simulink model "bit32alu"  (R2020a)
settings: Solver=VariableStepAuto  StartTime=0.0  StopTime=10.0  RelTol=1e-3
(part 1 of 62)
settings Model: Creator=kishan  LastModifiedBy=kishan

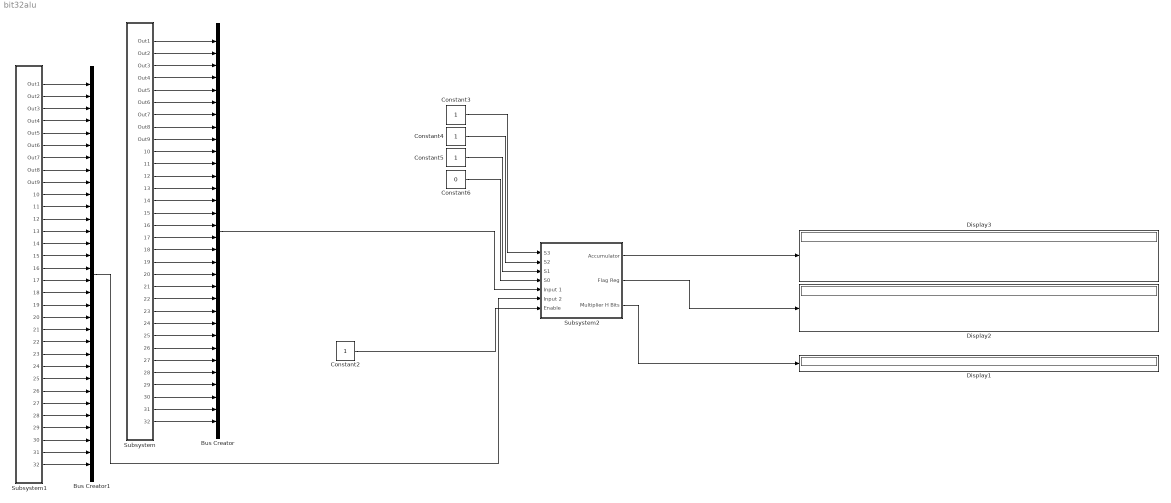
== system bit32alu ==
  Bus Creator : BusCreator  Inputs=32
  Bus Creator1 : BusCreator  Inputs=32
  Constant{2..5} (4 alike) : Constant  OutDataTypeStr=boolean
  Constant6 : Constant  Value=0  OutDataTypeStr=boolean
  Display1 : Display
  Display2 : Display
  Display3 : Display
  Subsystem : Subsystem
  Subsystem1 : Subsystem
  Subsystem2 : Subsystem
  wires:
  Subsystem/2(Out2) -> Bus Creator/2
  Subsystem/30(Out30) -> Bus Creator/30
  Subsystem/31(Out31) -> Bus Creator/31
  Subsystem/11(Out11) -> Bus Creator/11
  Subsystem/26(Out26) -> Bus Creator/26
  Subsystem/9(Out9) -> Bus Creator/9
  Subsystem/17(Out17) -> Bus Creator/17
  Subsystem/27(Out27) -> Bus Creator/27
  Subsystem/32(Out32) -> Bus Creator/32
  Subsystem/7(Out7) -> Bus Creator/7
  Subsystem/16(Out16) -> Bus Creator/16
  Subsystem/25(Out25) -> Bus Creator/25
  Subsystem/15(Out15) -> Bus Creator/15
  Subsystem/22(Out22) -> Bus Creator/22
  Subsystem/23(Out23) -> Bus Creator/23
  Subsystem/10(Out10) -> Bus Creator/10
  Subsystem/12(Out12) -> Bus Creator/12
  Subsystem/13(Out13) -> Bus Creator/13
  Subsystem/20(Out20) -> Bus Creator/20
  Subsystem/29(Out29) -> Bus Creator/29
  Subsystem/3(Out3) -> Bus Creator/3
  Subsystem/4(Out4) -> Bus Creator/4
  Subsystem/6(Out6) -> Bus Creator/6
  Subsystem/24(Out24) -> Bus Creator/24
  Subsystem/18(Out18) -> Bus Creator/18
  Subsystem/1(Out1) -> Bus Creator/1
  Subsystem/28(Out28) -> Bus Creator/28
  Subsystem/14(Out14) -> Bus Creator/14
  Subsystem/8(Out8) -> Bus Creator/8
  Subsystem/5(Out5) -> Bus Creator/5
  Subsystem/21(Out21) -> Bus Creator/21
  Subsystem/19(Out19) -> Bus Creator/19
  Subsystem1/2(Out2) -> Bus Creator1/2
  Subsystem1/30(Out30) -> Bus Creator1/30
  Subsystem1/31(Out31) -> Bus Creator1/31
  Subsystem1/11(Out11) -> Bus Creator1/11
  Subsystem1/26(Out26) -> Bus Creator1/26
  Subsystem1/9(Out9) -> Bus Creator1/9
  Subsystem1/17(Out17) -> Bus Creator1/17
  Subsystem1/27(Out27) -> Bus Creator1/27
  Subsystem1/32(Out32) -> Bus Creator1/32
  Subsystem1/7(Out7) -> Bus Creator1/7
  Subsystem1/16(Out16) -> Bus Creator1/16
  Subsystem1/25(Out25) -> Bus Creator1/25
  Subsystem1/15(Out15) -> Bus Creator1/15
  Subsystem1/22(Out22) -> Bus Creator1/22
  Subsystem1/23(Out23) -> Bus Creator1/23
  Subsystem1/10(Out10) -> Bus Creator1/10
  Subsystem1/12(Out12) -> Bus Creator1/12
  Subsystem1/13(Out13) -> Bus Creator1/13
  Subsystem1/20(Out20) -> Bus Creator1/20
  Subsystem1/29(Out29) -> Bus Creator1/29
  Subsystem1/3(Out3) -> Bus Creator1/3
  Subsystem1/4(Out4) -> Bus Creator1/4
  Subsystem1/6(Out6) -> Bus Creator1/6
  Subsystem1/24(Out24) -> Bus Creator1/24
  Subsystem1/18(Out18) -> Bus Creator1/18
  Subsystem1/1(Out1) -> Bus Creator1/1
  Subsystem1/28(Out28) -> Bus Creator1/28
  Subsystem1/14(Out14) -> Bus Creator1/14
  Subsystem1/8(Out8) -> Bus Creator1/8
  Subsystem1/5(Out5) -> Bus Creator1/5
  Subsystem1/21(Out21) -> Bus Creator1/21
  Subsystem1/19(Out19) -> Bus Creator1/19
  Constant3/1 -> Subsystem2/1(S3)
  Constant4/1 -> Subsystem2/2(S2)
  Constant5/1 -> Subsystem2/3(S1)
  Constant6/1 -> Subsystem2/4(S0)
  Bus Creator/1 -> Subsystem2/5(Input 1)
  Bus Creator1/1 -> Subsystem2/6(Input 2)
  Constant2/1 -> Subsystem2/7(Enable)
  Subsystem2/1(Accumulator) -> Display3/1
  Subsystem2/2(Flag Reg) -> Display2/1
  Subsystem2/3(Multiplier H Bits) -> Display1/1

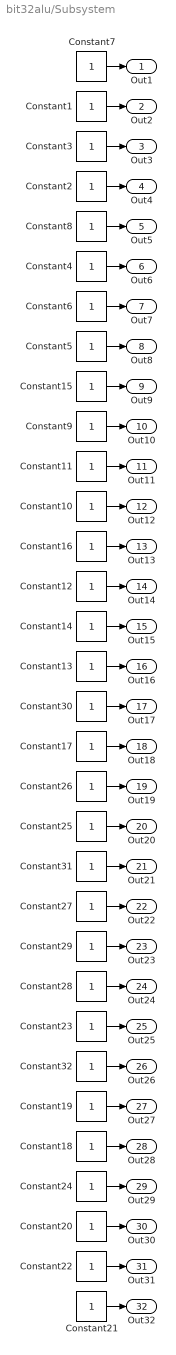
== system bit32alu/Subsystem ==
  Constant{1..32} (32 alike) : Constant  OutDataTypeStr=boolean
  Out1 : Outport
  Out2 : Outport  Port=2
  Out3 : Outport  Port=3
  Out4 : Outport  Port=4
  Out5 : Outport  Port=5
  Out6 : Outport  Port=6
  Out7 : Outport  Port=7
  Out8 : Outport  Port=8
  Out9 : Outport  Port=9
  Out10 : Outport  Port=10
  Out11 : Outport  Port=11
  Out12 : Outport  Port=12
  Out13 : Outport  Port=13
  Out14 : Outport  Port=14
  Out15 : Outport  Port=15
  Out16 : Outport  Port=16
  Out17 : Outport  Port=17
  Out18 : Outport  Port=18
  Out19 : Outport  Port=19
  Out20 : Outport  Port=20
  Out21 : Outport  Port=21
  Out22 : Outport  Port=22
  Out23 : Outport  Port=23
  Out24 : Outport  Port=24
  Out25 : Outport  Port=25
  Out26 : Outport  Port=26
  Out27 : Outport  Port=27
  Out28 : Outport  Port=28
  Out29 : Outport  Port=29
  Out30 : Outport  Port=30
  Out31 : Outport  Port=31
  Out32 : Outport  Port=32
  wires:
  Constant7/1 -> Out1/1
  Constant1/1 -> Out2/1
  Constant3/1 -> Out3/1
  Constant2/1 -> Out4/1
  Constant8/1 -> Out5/1
  Constant5/1 -> Out8/1
  Constant4/1 -> Out6/1
  Constant6/1 -> Out7/1
  Constant15/1 -> Out9/1
  Constant13/1 -> Out16/1
  Constant12/1 -> Out14/1
  Constant16/1 -> Out13/1
  Constant10/1 -> Out12/1
  Constant9/1 -> Out10/1
  Constant14/1 -> Out15/1
  Constant11/1 -> Out11/1
  Constant24/1 -> Out29/1
  Constant23/1 -> Out25/1
  Constant19/1 -> Out27/1
  Constant25/1 -> Out20/1
  Constant31/1 -> Out21/1
  Constant30/1 -> Out17/1
  Constant22/1 -> Out31/1
  Constant28/1 -> Out24/1
  Constant29/1 -> Out23/1
  Constant27/1 -> Out22/1
  Constant21/1 -> Out32/1
  Constant26/1 -> Out19/1
  Constant18/1 -> Out28/1
  Constant17/1 -> Out18/1
  Constant20/1 -> Out30/1
  Constant32/1 -> Out26/1

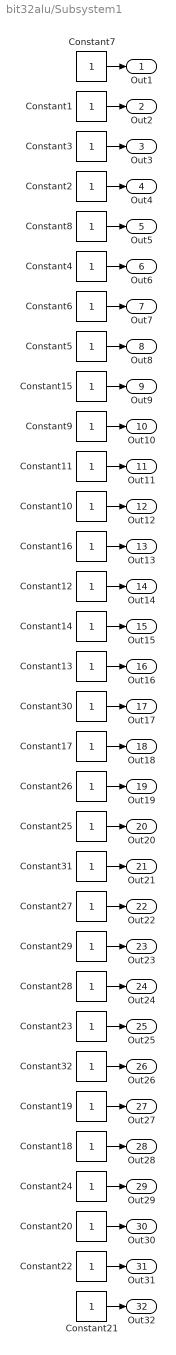
== system bit32alu/Subsystem1 ==
  Constant{1..32} (32 alike) : Constant  OutDataTypeStr=boolean
  Out1 : Outport
  Out2 : Outport  Port=2
  Out3 : Outport  Port=3
  Out4 : Outport  Port=4
  Out5 : Outport  Port=5
  Out6 : Outport  Port=6
  Out7 : Outport  Port=7
  Out8 : Outport  Port=8
  Out9 : Outport  Port=9
  Out10 : Outport  Port=10
  Out11 : Outport  Port=11
  Out12 : Outport  Port=12
  Out13 : Outport  Port=13
  Out14 : Outport  Port=14
  Out15 : Outport  Port=15
  Out16 : Outport  Port=16
  Out17 : Outport  Port=17
  Out18 : Outport  Port=18
  Out19 : Outport  Port=19
  Out20 : Outport  Port=20
  Out21 : Outport  Port=21
  Out22 : Outport  Port=22
  Out23 : Outport  Port=23
  Out24 : Outport  Port=24
  Out25 : Outport  Port=25
  Out26 : Outport  Port=26
  Out27 : Outport  Port=27
  Out28 : Outport  Port=28
  Out29 : Outport  Port=29
  Out30 : Outport  Port=30
  Out31 : Outport  Port=31
  Out32 : Outport  Port=32
  wires:
  Constant7/1 -> Out1/1
  Constant1/1 -> Out2/1
  Constant3/1 -> Out3/1
  Constant2/1 -> Out4/1
  Constant8/1 -> Out5/1
  Constant5/1 -> Out8/1
  Constant4/1 -> Out6/1
  Constant6/1 -> Out7/1
  Constant15/1 -> Out9/1
  Constant13/1 -> Out16/1
  Constant12/1 -> Out14/1
  Constant16/1 -> Out13/1
  Constant10/1 -> Out12/1
  Constant9/1 -> Out10/1
  Constant14/1 -> Out15/1
  Constant11/1 -> Out11/1
  Constant24/1 -> Out29/1
  Constant23/1 -> Out25/1
  Constant19/1 -> Out27/1
  Constant25/1 -> Out20/1
  Constant31/1 -> Out21/1
  Constant30/1 -> Out17/1
  Constant22/1 -> Out31/1
  Constant28/1 -> Out24/1
  Constant29/1 -> Out23/1
  Constant27/1 -> Out22/1
  Constant21/1 -> Out32/1
  Constant26/1 -> Out19/1
  Constant18/1 -> Out28/1
  Constant17/1 -> Out18/1
  Constant20/1 -> Out30/1
  Constant32/1 -> Out26/1

== system bit32alu/Subsystem2 ==
  S3 : Inport
  S2 : Inport  Port=2
  S1 : Inport  Port=3
  S0 : Inport  Port=4
  Input 1 : Inport  Port=5
  Input 2 : Inport  Port=6
  Enable : Inport  Port=7
  Adder : Subsystem
  Comparartor : Subsystem
  Decrementer : Subsystem
  Demux : Demux  Outputs=32
  Demux1 : Demux  Outputs=32
  Incrementer : Subsystem
  Left Rotator : Subsystem
  Left shifter : Subsystem
  Logical Operator : Logic  AllPortsSameDT=off  OutDataTypeStr=boolean
  Logical Operator1 : Logic  Operator=OR  AllPortsSameDT=off  OutDataTypeStr=boolean
  Logical Operator2 : Logic  Operator=NOT  AllPortsSameDT=off  OutDataTypeStr=boolean
  Logical Operator4 : Logic  Operator=NOR  Inputs=32  AllPortsSameDT=off  OutDataTypeStr=boolean
  Logical Operator5 : Logic  Operator=NXOR  Inputs=32  AllPortsSameDT=off  OutDataTypeStr=boolean
  Multiplier : Subsystem
  Mux : Mux  Inputs=8
  Ones : Constant  Value=[1 1 1 1 1 1 1 1 1 1 1 1 1 1 1 1 1 1 1 1 1 1 1 1 1 1 1 1 1 1 1 1]  OutDataTypeStr=boolean
  Right Shifter : Subsystem
  Right rotator : Subsystem
  Subsystem7 : Subsystem
  Subtractor : Subsystem
  Zeros : Constant  Value=[0 0 0 0 0 0 0 0 0 0 0 0 0 0 0 0 0 0 0 0 0 0 0 0 0 0 0 0 0 0 0 0]  OutDataTypeStr=boolean
  Accumulator : Outport
  Flag Reg : Outport  Port=2
  Multiplier H Bits : Outport  Port=3
  wires:
  Demux1/11 -> Logical Operator5/11
  Demux/9 -> Logical Operator4/9
  Demux/26 -> Logical Operator4/26
  Demux1/3 -> Logical Operator5/3
  Demux/12 -> Logical Operator4/12
  Demux1/16 -> Logical Operator5/16
  Demux/32 -> Logical Operator4/32
  Demux/14 -> Logical Operator4/14
  Demux/28 -> Logical Operator4/28
  Demux1/14 -> Logical Operator5/14
  Left Rotator/1(Out4) -> Subsystem7/17(In17)
  Demux1/13 -> Logical Operator5/13
  Demux/2 -> Logical Operator4/2
  S2/1 -> Subsystem7/2(In3)
  Right Shifter/2(Out4) -> Subsystem7/13(In13)
  Enable/1 -> Subsystem7/21(In21)
  Demux1/22 -> Logical Operator5/22
  Demux1/32 -> Logical Operator5/32
  Demux1/6 -> Logical Operator5/6
  Comparartor/1(Out1) -> Subsystem7/20(In20)
  Demux1/18 -> Logical Operator5/18
  Subsystem7/1(Out1) -> Accumulator/1, Demux1/1, Demux/1
  Demux/5 -> Logical Operator4/5
  Logical Operator1/1 -> Subsystem7/8(In6)
  Demux/11 -> Logical Operator4/11
  S3/1 -> Subsystem7/1(In1)
  Mux/1 -> Flag Reg/1
  Adder/1(Out1) -> Mux/5
  Logical Operator/1 -> Subsystem7/7(In4)
  Demux/31 -> Logical Operator4/31
  Logical Operator4/1 -> Mux/7
  Demux1/30 -> Logical Operator5/30
  Subtractor/1(Out1) -> Mux/6
  Demux/23 -> Logical Operator4/23
  Ones/1 -> Subsystem7/6(In2)
  Logical Operator5/1 -> Mux/8
  Demux/22 -> Logical Operator4/22
  Adder/2(Out2) -> Subsystem7/14(In14)
  Subtractor/2(Out2) -> Subsystem7/15(In15)
  Decrementer/2(Out2) -> Subsystem7/12(In12)
  Demux1/17 -> Logical Operator5/17
  Demux/6 -> Logical Operator4/6
  Demux/4 -> Logical Operator4/4
  Right rotator/1(Out2) -> Subsystem7/18(In18)
  Demux1/9 -> Logical Operator5/9
  Right Shifter/1(Out3) -> Mux/4
  Demux/17 -> Logical Operator4/17
  Demux/15 -> Logical Operator4/15
  Demux/7 -> Logical Operator4/7
  Demux1/2 -> Logical Operator5/2
  Demux1/5 -> Logical Operator5/5
  Demux1/31 -> Logical Operator5/31
  Zeros/1 -> Subsystem7/5(In9)
  Input 1/1 -> Left Rotator/1(Input 1), Right rotator/1(Input 1), Comparartor/1(In1), Adder/1(In1), Subsystem7/16(Input 1), Left shifter/1(Input 1), Right Shifter/1(Input 1), Decrementer/1(In1), Incrementer/1(In1), Logical Operator2/1, Logical Operator/1, Logical Operator1/1, Subtractor/1(In1), Multiplier/1(In1)
  Multiplier/2(Out2) -> Subsystem7/19(In19)
  Left shifter/1(Out1) -> Mux/2
  Demux1/27 -> Logical Operator5/27
  Demux/30 -> Logical Operator4/30
  Demux1/21 -> Logical Operator5/21
  Demux/18 -> Logical Operator4/18
  Demux/21 -> Logical Operator4/21
  Demux1/20 -> Logical Operator5/20
  Demux1/28 -> Logical Operator5/28
  Demux1/10 -> Logical Operator5/10
  Demux1/25 -> Logical Operator5/25
  Demux/29 -> Logical Operator4/29
  Incrementer/2(Out2) -> Subsystem7/10(In10)
  Left shifter/2(Out2) -> Subsystem7/11(In11)
  Demux/20 -> Logical Operator4/20
  Demux1/19 -> Logical Operator5/19
  Demux1/8 -> Logical Operator5/8
  Demux/25 -> Logical Operator4/25
  Demux1/1 -> Logical Operator5/1
  Demux1/15 -> Logical Operator5/15
  Demux1/23 -> Logical Operator5/23
  Multiplier/1(Out1) -> Multiplier H Bits/1
  Demux/8 -> Logical Operator4/8
  Demux/1 -> Logical Operator4/1
  Demux1/26 -> Logical Operator5/26
  Demux1/24 -> Logical Operator5/24
  S0/1 -> Subsystem7/4(In7)
  Logical Operator2/1 -> Subsystem7/9(In8)
  Demux/10 -> Logical Operator4/10
  Demux/24 -> Logical Operator4/24
  Decrementer/1(Out1) -> Mux/3
  Demux1/4 -> Logical Operator5/4
  Demux/16 -> Logical Operator4/16
  Demux1/12 -> Logical Operator5/12
  Demux/3 -> Logical Operator4/3
  Incrementer/1(Out1) -> Mux/1
  Demux1/7 -> Logical Operator5/7
  Demux/13 -> Logical Operator4/13
  Input 2/1 -> Comparartor/2(In2), Logical Operator1/2, Logical Operator/2, Subtractor/2(In2), Adder/2(In2), Multiplier/2(In2)
  Demux/19 -> Logical Operator4/19
  Demux/27 -> Logical Operator4/27
  S1/1 -> Subsystem7/3(In5)
  Demux1/29 -> Logical Operator5/29

== system bit32alu/Subsystem2/Adder ==
  In1 : Inport
  In2 : Inport  Port=2
  Subsystem : Subsystem
  Zeros1 : Constant  Value=0  OutDataTypeStr=boolean
  Out1 : Outport
  Out2 : Outport  Port=2
  wires:
  Subsystem/2(Out2) -> Out2/1
  In2/1 -> Subsystem/3(In3)
  Zeros1/1 -> Subsystem/2(In2)
  In1/1 -> Subsystem/1(In1)
  Subsystem/1(Out1) -> Out1/1

== system bit32alu/Subsystem2/Comparartor ==
  In1 : Inport
  In2 : Inport  Port=2
  Comparator : Subsystem
  Comparator1 : Subsystem
  Comparator2 : Subsystem
  Comparator3 : Subsystem
  Demux : Demux
  Demux1 : Demux
  Display : Display
  Logical Operator : Logic  Operator=OR  Inputs=4  AllPortsSameDT=off  OutDataTypeStr=boolean
  Logical Operator1 : Logic  Inputs=4  AllPortsSameDT=off  OutDataTypeStr=boolean
  Logical Operator2 : Logic  AllPortsSameDT=off  OutDataTypeStr=boolean
  Logical Operator3 : Logic  Inputs=3  AllPortsSameDT=off  OutDataTypeStr=boolean
  Logical Operator4 : Logic  Inputs=4  AllPortsSameDT=off  OutDataTypeStr=boolean
  Logical Operator5 : Logic  Operator=NOR  AllPortsSameDT=off  OutDataTypeStr=boolean
  Mux : Mux
  Mux1 : Mux
  Zeros1 : Constant  Value=[0 0 0 0 0 0 0 0 0 0 0 0 0 0 0 0 0 0 0 0 0 0 0 0 0 0 0 0 0]  OutDataTypeStr=boolean
  Out1 : Outport
  wires:
  Zeros1/1 -> Mux/4
  Mux/1 -> Out1/1
  In1/1 -> Demux/1
  In2/1 -> Demux1/1
  Demux/1 -> Comparator/1(In1)
  Demux/2 -> Comparator1/1(In1)
  Demux/3 -> Comparator2/1(In1)
  Demux/4 -> Comparator3/1(In1)
  Demux1/1 -> Comparator/2(In2)
  Demux1/2 -> Comparator1/2(In2)
  Demux1/3 -> Comparator2/2(In2)
  Demux1/4 -> Comparator3/2(In2)
  Comparator/2(Out2) -> Logical Operator1/1, Logical Operator4/1, Logical Operator3/1, Logical Operator2/1
  Comparator1/2(Out2) -> Logical Operator4/2, Logical Operator3/2, Logical Operator1/2
  Comparator2/2(Out2) -> Logical Operator4/3, Logical Operator1/3
  Comparator3/2(Out2) -> Logical Operator1/4
  Logical Operator1/1 -> Logical Operator5/2, Mux/2
  Mux1/1 -> Display/1
  Comparator/1(Out1) -> Logical Operator/1
  Comparator1/1(Out1) -> Logical Operator2/2
  Logical Operator2/1 -> Logical Operator/2
  Comparator2/1(Out1) -> Logical Operator3/3
  Logical Operator3/1 -> Logical Operator/3
  Comparator3/1(Out1) -> Logical Operator4/4
  Logical Operator4/1 -> Logical Operator/4
  Logical Operator/1 -> Logical Operator5/1, Mux/1
  Comparator/3(Out3) -> Mux1/1
  Comparator1/3(Out3) -> Mux1/2
  Comparator2/3(Out3) -> Mux1/3
  Comparator3/3(Out3) -> Mux1/4
  Logical Operator5/1 -> Mux/3

== system bit32alu/Subsystem2/Decrementer ==
  In1 : Inport
  Subtractor1 : Subsystem
  Zeros1 : Constant  Value=[0 0 0 0 0 0 0 0 0 0 0 0 0 0 0 0 0 0 0 0 0 0 0 0 0 0 0 0 0 0 0 1]
  Out1 : Outport
  Out2 : Outport  Port=2
  wires:
  Zeros1/1 -> Subtractor1/2(In2)
  In1/1 -> Subtractor1/1(In1)
  Subtractor1/1(Out1) -> Out1/1
  Subtractor1/2(Out2) -> Out2/1

== system bit32alu/Subsystem2/Incrementer ==
  In1 : Inport
  Incrementer : Subsystem
  Zeros1 : Constant  Value=[0 0 0 0 0 0 0 0 0 0 0 0 0 0 0 0 0 0 0 0 0 0 0 0 0 0 0 0 0 0 0 1]  OutDataTypeStr=boolean
  Out1 : Outport
  Out2 : Outport  Port=2
  wires:
  Zeros1/1 -> Incrementer/2(In2)
  In1/1 -> Incrementer/1(In1)
  Incrementer/2(Out2) -> Out2/1
  Incrementer/1(Out1) -> Out1/1

== system bit32alu/Subsystem2/Left Rotator ==
  Input 1 : Inport
  Demux : Demux  Outputs=32
  Mux : Mux  Inputs=32
  Out4 : Outport
  wires:
  Input 1/1 -> Demux/1
  Mux/1 -> Out4/1
  Demux/1 -> Mux/2
  Demux/2 -> Mux/3
  Demux/3 -> Mux/4
  Demux/4 -> Mux/5
  Demux/5 -> Mux/6
  Demux/6 -> Mux/7
  Demux/7 -> Mux/8
  Demux/8 -> Mux/9
  Demux/9 -> Mux/10
  Demux/10 -> Mux/11
  Demux/11 -> Mux/12
  Demux/12 -> Mux/13
  Demux/13 -> Mux/14
  Demux/14 -> Mux/15
  Demux/15 -> Mux/16
  Demux/16 -> Mux/17
  Demux/17 -> Mux/18
  Demux/18 -> Mux/19
  Demux/19 -> Mux/20
  Demux/20 -> Mux/21
  Demux/21 -> Mux/22
  Demux/22 -> Mux/23
  Demux/23 -> Mux/24
  Demux/24 -> Mux/25
  Demux/25 -> Mux/26
  Demux/26 -> Mux/27
  Demux/27 -> Mux/28
  Demux/28 -> Mux/29
  Demux/29 -> Mux/30
  Demux/30 -> Mux/31
  Demux/31 -> Mux/32
  Demux/32 -> Mux/1

== system bit32alu/Subsystem2/Left shifter ==
  Input 1 : Inport
  Demux : Demux  Outputs=32
  Mux : Mux  Inputs=32
  Zeros1 : Constant  Value=0  OutDataTypeStr=boolean
  Out1 : Outport
  Out2 : Outport  Port=2
  wires:
  Zeros1/1 -> Mux/32
  Input 1/1 -> Demux/1
  Mux/1 -> Out2/1
  Demux/1 -> Out1/1
  Demux/2 -> Mux/1
  Demux/3 -> Mux/2
  Demux/4 -> Mux/3
  Demux/5 -> Mux/4
  Demux/6 -> Mux/5
  Demux/7 -> Mux/6
  Demux/8 -> Mux/7
  Demux/9 -> Mux/8
  Demux/10 -> Mux/9
  Demux/11 -> Mux/10
  Demux/12 -> Mux/11
  Demux/13 -> Mux/12
  Demux/14 -> Mux/13
  Demux/15 -> Mux/14
  Demux/16 -> Mux/15
  Demux/17 -> Mux/16
  Demux/18 -> Mux/17
  Demux/19 -> Mux/18
  Demux/20 -> Mux/19
  Demux/21 -> Mux/20
  Demux/22 -> Mux/21
  Demux/23 -> Mux/22
  Demux/24 -> Mux/23
  Demux/25 -> Mux/24
  Demux/26 -> Mux/25
  Demux/27 -> Mux/26
  Demux/28 -> Mux/27
  Demux/29 -> Mux/28
  Demux/30 -> Mux/29
  Demux/31 -> Mux/30
  Demux/32 -> Mux/31

== system bit32alu/Subsystem2/Multiplier ==
  In1 : Inport
  In2 : Inport  Port=2
  Constant : Constant  Value=0  OutDataTypeStr=boolean
  Constant1 : Constant  Value=0  OutDataTypeStr=boolean
  Constant2 : Constant  Value=[0 0 0 0 0 0 0 0 0 0 0 0 0 0 0]  OutDataTypeStr=boolean
  Demux : Demux  Outputs=2
  Demux1 : Demux  Outputs=2
  Demux2 : Demux  Outputs=2
  Display : Display
  Logical Operator : Logic  AllPortsSameDT=off  OutDataTypeStr=boolean
  Logical Operator1 : Logic  Operator=XOR  AllPortsSameDT=off  OutDataTypeStr=boolean
  Mux{,1..3} (4 alike) : Mux  Inputs=2
  Mux4 : Mux  Inputs=3
  Subsystem : Subsystem
  Subsystem1 : Subsystem
  Subsystem2 : Subsystem
  Subsystem3 : Subsystem
  Subsystem4 : Subsystem
  Subsystem5 : Subsystem
  Subsystem7 : Subsystem
  Out1 : Outport
  Out2 : Outport  Port=2
  wires:
  Constant1/1 -> Subsystem4/2(In2)
  Subsystem3/1(Out1) -> Mux2/2
  Logical Operator/1 -> Subsystem5/2(In2)
  Subsystem3/2(Out2) -> Mux4/3
  Subsystem5/2(Out2) -> Mux4/1
  Demux/2 -> Subsystem3/1(In1), Subsystem2/1(In1)
  Mux1/1 -> Subsystem/3(In3)
  Mux3/1 -> Subsystem5/3(In3)
  Subsystem4/1(Out1) -> Logical Operator/2, Logical Operator1/2
  Logical Operator1/1 -> Mux3/2
  Subsystem2/1(Out1) -> Mux1/1
  Subsystem/1(Out1) -> Logical Operator/1, Logical Operator1/1
  Subsystem5/1(Out1) -> Display/1
  In1/1 -> Demux/1
  Demux1/2 -> Subsystem1/2(In2), Subsystem3/2(In2)
  Constant/1 -> Subsystem/2(In2)
  Subsystem7/1(Out1) -> Subsystem5/1(In1)
  In2/1 -> Demux1/1
  Subsystem7/2(Out2) -> Mux2/1
  Subsystem4/2(Out2) -> Mux4/2
  Subsystem/2(Out2) -> Subsystem4/1(In1)
  Demux/1 -> Subsystem1/1(In1), Subsystem7/1(In1)
  Subsystem1/2(Out2) -> Mux/2
  Demux1/1 -> Subsystem7/2(In2), Subsystem2/2(In2)
  Constant2/1 -> Mux3/1
  Subsystem2/2(Out2) -> Mux1/2
  Mux/1 -> Subsystem/1(In1)
  Mux2/1 -> Subsystem4/3(In3)
  Subsystem1/1(Out1) -> Mux/1
  Mux4/1 -> Demux2/1
  Demux2/1 -> Out1/1
  Demux2/2 -> Out2/1

== system bit32alu/Subsystem2/Right Shifter ==
  Input 1 : Inport
  Demux : Demux  Outputs=32
  Mux : Mux  Inputs=32
  Zeros2 : Constant  Value=0  OutDataTypeStr=boolean
  Out3 : Outport
  Out4 : Outport  Port=2
  wires:
  Input 1/1 -> Demux/1
  Mux/1 -> Out4/1
  Demux/1 -> Mux/2
  Demux/2 -> Mux/3
  Demux/3 -> Mux/4
  Demux/4 -> Mux/5
  Demux/5 -> Mux/6
  Demux/6 -> Mux/7
  Demux/7 -> Mux/8
  Demux/8 -> Mux/9
  Demux/9 -> Mux/10
  Demux/10 -> Mux/11
  Demux/11 -> Mux/12
  Demux/12 -> Mux/13
  Demux/13 -> Mux/14
  Demux/14 -> Mux/15
  Demux/15 -> Mux/16
  Demux/16 -> Mux/17
  Demux/17 -> Mux/18
  Demux/18 -> Mux/19
  Demux/19 -> Mux/20
  Demux/20 -> Mux/21
  Demux/21 -> Mux/22
  Demux/22 -> Mux/23
  Demux/23 -> Mux/24
  Demux/24 -> Mux/25
  Demux/25 -> Mux/26
  Demux/26 -> Mux/27
  Demux/27 -> Mux/28
  Demux/28 -> Mux/29
  Demux/29 -> Mux/30
  Demux/30 -> Mux/31
  Demux/31 -> Mux/32
  Zeros2/1 -> Mux/1
  Demux/32 -> Out3/1

== system bit32alu/Subsystem2/Right rotator ==
  Input 1 : Inport
  Demux : Demux  Outputs=32
  Mux : Mux  Inputs=32
  Out2 : Outport
  wires:
  Input 1/1 -> Demux/1
  Mux/1 -> Out2/1
  Demux/2 -> Mux/1
  Demux/3 -> Mux/2
  Demux/4 -> Mux/3
  Demux/5 -> Mux/4
  Demux/6 -> Mux/5
  Demux/7 -> Mux/6
  Demux/8 -> Mux/7
  Demux/9 -> Mux/8
  Demux/10 -> Mux/9
  Demux/11 -> Mux/10
  Demux/12 -> Mux/11
  Demux/13 -> Mux/12
  Demux/14 -> Mux/13
  Demux/15 -> Mux/14
  Demux/16 -> Mux/15
  Demux/17 -> Mux/16
  Demux/18 -> Mux/17
  Demux/19 -> Mux/18
  Demux/20 -> Mux/19
  Demux/21 -> Mux/20
  Demux/22 -> Mux/21
  Demux/23 -> Mux/22
  Demux/24 -> Mux/23
  Demux/25 -> Mux/24
  Demux/26 -> Mux/25
  Demux/27 -> Mux/26
  Demux/28 -> Mux/27
  Demux/29 -> Mux/28
  Demux/30 -> Mux/29
  Demux/31 -> Mux/30
  Demux/32 -> Mux/31
  Demux/1 -> Mux/32

== system bit32alu/Subsystem2/Subsystem7 ==
  In1 : Inport
  In3 : Inport  Port=2
  In5 : Inport  Port=3
  In7 : Inport  Port=4
  In9 : Inport  Port=5
  In2 : Inport  Port=6
  In4 : Inport  Port=7
  In6 : Inport  Port=8
  In8 : Inport  Port=9
  In10 : Inport  Port=10
  In11 : Inport  Port=11
  In12 : Inport  Port=12
  In13 : Inport  Port=13
  In14 : Inport  Port=14
  In15 : Inport  Port=15
  Input 1 : Inport  Port=16
  In17 : Inport  Port=17
  In18 : Inport  Port=18
  In19 : Inport  Port=19
  In20 : Inport  Port=20
  In21 : Inport  Port=21
  Demux{,1..15} (16 alike) : Demux
  Mux : Mux
  Subsystem1 : Subsystem
  Subsystem2 : Subsystem
  Subsystem3 : Subsystem
  Subsystem4 : Subsystem
  Out1 : Outport
  wires:
  In3/1 -> Subsystem3/2(In21), Subsystem4/2(In21), Subsystem2/2(In21), Subsystem1/2(In21)
  In7/1 -> Subsystem4/4(In2), Subsystem3/4(In2), Subsystem2/4(In2), Subsystem1/4(In2)
  Subsystem3/1(Out1) -> Mux/1
  Subsystem4/1(Out1) -> Mux/2
  Subsystem2/1(Out1) -> Mux/4
  In5/1 -> Subsystem4/3(In1), Subsystem3/3(In1), Subsystem2/3(In1), Subsystem1/3(In1)
  In1/1 -> Subsystem4/1(In20), Subsystem3/1(In20), Subsystem2/1(In20), Subsystem1/1(In20)
  Subsystem1/1(Out1) -> Mux/3
  Mux/1 -> Out1/1
  In9/1 -> Demux/1
  In21/1 -> Subsystem4/21(In19), Subsystem3/21(In19), Subsystem2/21(In19), Subsystem1/21(In19)
  Demux/1 -> Subsystem3/5(In3)
  Demux/2 -> Subsystem4/5(In3)
  Demux/3 -> Subsystem1/5(In3)
  Demux/4 -> Subsystem2/5(In3)
  Demux1/4 -> Subsystem2/6(In4)
  Demux1/1 -> Subsystem3/6(In4)
  Demux1/2 -> Subsystem4/6(In4)
  Demux1/3 -> Subsystem1/6(In4)
  In2/1 -> Demux1/1
  Demux2/2 -> Subsystem4/7(In5)
  Demux3/1 -> Subsystem3/8(In6)
  Demux2/3 -> Subsystem1/7(In5)
  Demux3/2 -> Subsystem4/8(In6)
  Demux2/4 -> Subsystem2/7(In5)
  In6/1 -> Demux3/1
  Demux2/1 -> Subsystem3/7(In5)
  Demux3/3 -> Subsystem1/8(In6)
  Demux3/4 -> Subsystem2/8(In6)
  In4/1 -> Demux2/1
  In10/1 -> Demux5/1
  In11/1 -> Demux6/1
  Demux6/3 -> Subsystem1/11(In9)
  Demux4/2 -> Subsystem4/9(In7)
  Demux7/2 -> Subsystem4/12(In10)
  Demux5/1 -> Subsystem3/10(In8)
  Demux5/2 -> Subsystem4/10(In8)
  Demux4/3 -> Subsystem1/9(In7)
  Demux4/4 -> Subsystem2/9(In7)
  Demux6/4 -> Subsystem2/11(In9)
  Demux7/1 -> Subsystem3/12(In10)
  Demux6/2 -> Subsystem4/11(In9)
  Demux7/4 -> Subsystem2/12(In10)
  Demux4/1 -> Subsystem3/9(In7)
  Demux6/1 -> Subsystem3/11(In9)
  Demux5/4 -> Subsystem2/10(In8)
  Demux5/3 -> Subsystem1/10(In8)
  Demux7/3 -> Subsystem1/12(In10)
  In12/1 -> Demux7/1
  In8/1 -> Demux4/1
  Demux11/4 -> Subsystem2/16(In14)
  Demux15/1 -> Subsystem3/20(In18)
  Demux10/2 -> Subsystem4/15(In13)
  In20/1 -> Demux15/1
  Demux8/2 -> Subsystem4/13(In11)
  Demux12/4 -> Subsystem2/17(In15)
  Demux13/1 -> Subsystem3/18(In16)
  Demux13/4 -> Subsystem2/18(In16)
  Demux11/3 -> Subsystem1/16(In14)
  Demux15/4 -> Subsystem2/20(In18)
  Demux10/4 -> Subsystem2/15(In13)
  Demux15/3 -> Subsystem1/20(In18)
  In14/1 -> Demux9/1
  Demux9/4 -> Subsystem2/14(In12)
  Demux14/4 -> Subsystem2/19(In17)
  Demux12/2 -> Subsystem4/17(In15)
  Demux8/3 -> Subsystem1/13(In11)
  Demux15/2 -> Subsystem4/20(In18)
  Demux9/2 -> Subsystem4/14(In12)
  In15/1 -> Demux10/1
  Demux11/2 -> Subsystem4/16(In14)
  Demux14/1 -> Subsystem3/19(In17)
  Demux12/1 -> Subsystem3/17(In15)
  Demux10/3 -> Subsystem1/15(In13)
  Demux12/3 -> Subsystem1/17(In15)
  Demux13/2 -> Subsystem4/18(In16)
  Demux9/1 -> Subsystem3/14(In12)
  Demux11/1 -> Subsystem3/16(In14)
  Demux8/1 -> Subsystem3/13(In11)
  Demux14/3 -> Subsystem1/19(In17)
  Demux14/2 -> Subsystem4/19(In17)
  Demux13/3 -> Subsystem1/18(In16)
  Demux8/4 -> Subsystem2/13(In11)
  Demux10/1 -> Subsystem3/15(In13)
  In19/1 -> Demux14/1
  Demux9/3 -> Subsystem1/14(In12)
  In18/1 -> Demux13/1
  Input 1/1 -> Demux11/1
  In17/1 -> Demux12/1
  In13/1 -> Demux8/1

== system bit32alu/Subsystem2/Subtractor ==
  In1 : Inport
  In2 : Inport  Port=2
  Logical Operator2 : Logic  Operator=NOT  AllPortsSameDT=off  OutDataTypeStr=boolean
  Subtractor : Subsystem
  Zeros1 : Constant  OutDataTypeStr=boolean
  Out1 : Outport
  Out2 : Outport  Port=2
  wires:
  In2/1 -> Logical Operator2/1
  Subtractor/1(Out1) -> Out1/1
  In1/1 -> Subtractor/1(In1)
  Subtractor/2(Out2) -> Out2/1
  Logical Operator2/1 -> Subtractor/3(In3)
  Zeros1/1 -> Subtractor/2(In2)

== system bit32alu/Subsystem2/Adder/Subsystem ==
  In1 : Inport
  In2 : Inport  Port=2
  In3 : Inport  Port=3
  Demux : Demux  Outputs=2
  Demux1 : Demux  Outputs=2
  Mux : Mux  Inputs=2
  Subsystem1 : Subsystem
  Subsystem2 : Subsystem
  Out1 : Outport
  Out2 : Outport  Port=2
  wires:
  Mux/1 -> Out2/1
  In3/1 -> Demux1/1
  Subsystem2/2(Out2) -> Mux/2
  In1/1 -> Demux/1
  Subsystem2/1(Out1) -> Subsystem1/2(In2)
  Subsystem1/2(Out2) -> Mux/1
  Demux1/2 -> Subsystem2/3(In3)
  In2/1 -> Subsystem2/2(In2)
  Demux/2 -> Subsystem2/1(In1)
  Subsystem1/1(Out1) -> Out1/1
  Demux1/1 -> Subsystem1/3(In3)
  Demux/1 -> Subsystem1/1(In1)

== system bit32alu/Subsystem2/Comparartor/Comparator ==
  In1 : Inport
  In2 : Inport  Port=2
  Demux{,1..3} (4 alike) : Demux  Outputs=8
  Logical Operator{1..3,7,9..12,14..15,17..18,21,23..24} (15 alike) : Logic  Operator=NOT  Inputs=3  AllPortsSameDT=off  OutDataTypeStr=boolean
  Logical Operator{4,8,13,16,19..20,22} (7 alike) : Logic  Inputs=3  AllPortsSameDT=off  OutDataTypeStr=boolean
  Logical Operator25 : Logic  Operator=NOR  AllPortsSameDT=off  OutDataTypeStr=boolean
  Logical Operator5 : Logic  AllPortsSameDT=off  OutDataTypeStr=boolean
  Logical Operator6 : Logic  Operator=OR  Inputs=8  AllPortsSameDT=off  OutDataTypeStr=boolean
  NOT{1..8} (8 alike) : Logic  Operator=NXOR  AllPortsSameDT=off  OutDataTypeStr=boolean
  NOT9 : Logic  Inputs=8  AllPortsSameDT=off  OutDataTypeStr=boolean
  Out1 : Outport
  Out2 : Outport  Port=2
  Out3 : Outport  Port=3
  wires:
  Demux/1 -> NOT1/1
  Demux/2 -> NOT2/1
  Demux/3 -> NOT3/1
  Demux/4 -> NOT4/1
  Demux/5 -> NOT5/1
  Demux/6 -> NOT6/1
  Demux/7 -> NOT7/1
  Demux/8 -> NOT8/1
  Demux1/1 -> NOT1/2
  Demux1/2 -> NOT2/2
  Demux1/3 -> NOT3/2
  Demux1/4 -> NOT4/2
  Demux1/5 -> NOT5/2
  Demux1/6 -> NOT6/2
  Demux1/7 -> NOT7/2
  Demux1/8 -> NOT8/2
  In1/1 -> Demux2/1, Demux/1
  In2/1 -> Demux1/1, Demux3/1
  NOT1/1 -> NOT9/1
  NOT2/1 -> NOT9/2
  NOT3/1 -> NOT9/3
  NOT4/1 -> NOT9/4
  NOT5/1 -> NOT9/5
  NOT6/1 -> NOT9/6
  NOT7/1 -> NOT9/7
  NOT8/1 -> NOT9/8
  NOT9/1 -> Logical Operator25/2, Out2/1
  Logical Operator14/1 -> Logical Operator16/3
  Logical Operator7/1 -> Logical Operator8/1
  Logical Operator13/1 -> Logical Operator15/1, Logical Operator6/3
  Demux3/1 -> Logical Operator9/1
  Demux2/2 -> Logical Operator8/2
  Logical Operator15/1 -> Logical Operator16/1
  Demux2/3 -> Logical Operator13/2
  Logical Operator10/1 -> Logical Operator8/3
  Logical Operator6/1 -> Logical Operator25/1, Out1/1
  Demux2/1 -> Logical Operator5/1
  Demux2/4 -> Logical Operator16/2
  Logical Operator11/1 -> Logical Operator13/3
  Logical Operator16/1 -> Logical Operator24/1, Logical Operator6/4
  Logical Operator9/1 -> Logical Operator5/2
  Demux3/2 -> Logical Operator10/1
  Logical Operator12/1 -> Logical Operator13/1
  Demux3/3 -> Logical Operator11/1
  Demux3/4 -> Logical Operator14/1
  Logical Operator5/1 -> Logical Operator7/1, Logical Operator6/1
  Logical Operator8/1 -> Logical Operator12/1, Logical Operator6/2
  Demux2/5 -> Logical Operator20/1
  Demux3/5 -> Logical Operator23/1
  Logical Operator17/1 -> Logical Operator19/3
  Logical Operator19/1 -> Logical Operator6/8
  Logical Operator1/1 -> Logical Operator22/3
  Logical Operator2/1 -> Logical Operator4/3
  Demux3/8 -> Logical Operator17/1
  Demux3/7 -> Logical Operator2/1
  Demux2/7 -> Logical Operator4/2
  Logical Operator3/1 -> Logical Operator4/1
  Logical Operator21/1 -> Logical Operator22/1
  Logical Operator22/1 -> Logical Operator6/6, Logical Operator3/1
  Demux2/8 -> Logical Operator19/2
  Logical Operator18/1 -> Logical Operator19/1
  Logical Operator20/1 -> Logical Operator6/5, Logical Operator21/1
  Demux3/6 -> Logical Operator1/1
  Logical Operator4/1 -> Logical Operator6/7, Logical Operator18/1
  Demux2/6 -> Logical Operator22/2
  Logical Operator24/1 -> Logical Operator20/2
  Logical Operator23/1 -> Logical Operator20/3
  Logical Operator25/1 -> Out3/1

== system bit32alu/Subsystem2/Comparartor/Comparator1 ==
  In1 : Inport
  In2 : Inport  Port=2
  Demux{,1..3} (4 alike) : Demux  Outputs=8
  Logical Operator{1..3,7,9..12,14..15,17..18,21,23..24} (15 alike) : Logic  Operator=NOT  Inputs=3  AllPortsSameDT=off  OutDataTypeStr=boolean
  Logical Operator{4,8,13,16,19..20,22} (7 alike) : Logic  Inputs=3  AllPortsSameDT=off  OutDataTypeStr=boolean
  Logical Operator25 : Logic  Operator=NOR  AllPortsSameDT=off  OutDataTypeStr=boolean
  Logical Operator5 : Logic  AllPortsSameDT=off  OutDataTypeStr=boolean
  Logical Operator6 : Logic  Operator=OR  Inputs=8  AllPortsSameDT=off  OutDataTypeStr=boolean
  NOT{1..8} (8 alike) : Logic  Operator=NXOR  AllPortsSameDT=off  OutDataTypeStr=boolean
  NOT9 : Logic  Inputs=8  AllPortsSameDT=off  OutDataTypeStr=boolean
  Out1 : Outport
  Out2 : Outport  Port=2
  Out3 : Outport  Port=3
  wires:
  Demux/1 -> NOT1/1
  Demux/2 -> NOT2/1
  Demux/3 -> NOT3/1
  Demux/4 -> NOT4/1
  Demux/5 -> NOT5/1
  Demux/6 -> NOT6/1
  Demux/7 -> NOT7/1
  Demux/8 -> NOT8/1
  Demux1/1 -> NOT1/2
  Demux1/2 -> NOT2/2
  Demux1/3 -> NOT3/2
  Demux1/4 -> NOT4/2
  Demux1/5 -> NOT5/2
  Demux1/6 -> NOT6/2
  Demux1/7 -> NOT7/2
  Demux1/8 -> NOT8/2
  In1/1 -> Demux2/1, Demux/1
  In2/1 -> Demux1/1, Demux3/1
  NOT1/1 -> NOT9/1
  NOT2/1 -> NOT9/2
  NOT3/1 -> NOT9/3
  NOT4/1 -> NOT9/4
  NOT5/1 -> NOT9/5
  NOT6/1 -> NOT9/6
  NOT7/1 -> NOT9/7
  NOT8/1 -> NOT9/8
  NOT9/1 -> Logical Operator25/2, Out2/1
  Logical Operator14/1 -> Logical Operator16/3
  Logical Operator7/1 -> Logical Operator8/1
  Logical Operator13/1 -> Logical Operator15/1, Logical Operator6/3
  Demux3/1 -> Logical Operator9/1
  Demux2/2 -> Logical Operator8/2
  Logical Operator15/1 -> Logical Operator16/1
  Demux2/3 -> Logical Operator13/2
  Logical Operator10/1 -> Logical Operator8/3
  Logical Operator6/1 -> Logical Operator25/1, Out1/1
  Demux2/1 -> Logical Operator5/1
  Demux2/4 -> Logical Operator16/2
  Logical Operator11/1 -> Logical Operator13/3
  Logical Operator16/1 -> Logical Operator24/1, Logical Operator6/4
  Logical Operator9/1 -> Logical Operator5/2
  Demux3/2 -> Logical Operator10/1
  Logical Operator12/1 -> Logical Operator13/1
  Demux3/3 -> Logical Operator11/1
  Demux3/4 -> Logical Operator14/1
  Logical Operator5/1 -> Logical Operator7/1, Logical Operator6/1
  Logical Operator8/1 -> Logical Operator12/1, Logical Operator6/2
  Demux2/5 -> Logical Operator20/1
  Demux3/5 -> Logical Operator23/1
  Logical Operator17/1 -> Logical Operator19/3
  Logical Operator19/1 -> Logical Operator6/8
  Logical Operator1/1 -> Logical Operator22/3
  Logical Operator2/1 -> Logical Operator4/3
  Demux3/8 -> Logical Operator17/1
  Demux3/7 -> Logical Operator2/1
  Demux2/7 -> Logical Operator4/2
  Logical Operator3/1 -> Logical Operator4/1
  Logical Operator21/1 -> Logical Operator22/1
  Logical Operator22/1 -> Logical Operator6/6, Logical Operator3/1
  Demux2/8 -> Logical Operator19/2
  Logical Operator18/1 -> Logical Operator19/1
  Logical Operator20/1 -> Logical Operator6/5, Logical Operator21/1
  Demux3/6 -> Logical Operator1/1
  Logical Operator4/1 -> Logical Operator6/7, Logical Operator18/1
  Demux2/6 -> Logical Operator22/2
  Logical Operator24/1 -> Logical Operator20/2
  Logical Operator23/1 -> Logical Operator20/3
  Logical Operator25/1 -> Out3/1

== system bit32alu/Subsystem2/Comparartor/Comparator2 ==
  In1 : Inport
  In2 : Inport  Port=2
  Demux{,1..3} (4 alike) : Demux  Outputs=8
  Logical Operator{1..3,7,9..12,14..15,17..18,21,23..24} (15 alike) : Logic  Operator=NOT  Inputs=3  AllPortsSameDT=off  OutDataTypeStr=boolean
  Logical Operator{4,8,13,16,19..20,22} (7 alike) : Logic  Inputs=3  AllPortsSameDT=off  OutDataTypeStr=boolean
  Logical Operator25 : Logic  Operator=NOR  AllPortsSameDT=off  OutDataTypeStr=boolean
  Logical Operator5 : Logic  AllPortsSameDT=off  OutDataTypeStr=boolean
  Logical Operator6 : Logic  Operator=OR  Inputs=8  AllPortsSameDT=off  OutDataTypeStr=boolean
  NOT{1..8} (8 alike) : Logic  Operator=NXOR  AllPortsSameDT=off  OutDataTypeStr=boolean
  NOT9 : Logic  Inputs=8  AllPortsSameDT=off  OutDataTypeStr=boolean
  Out1 : Outport
  Out2 : Outport  Port=2
  Out3 : Outport  Port=3
  wires:
  Demux/1 -> NOT1/1
  Demux/2 -> NOT2/1
  Demux/3 -> NOT3/1
  Demux/4 -> NOT4/1
  Demux/5 -> NOT5/1
  Demux/6 -> NOT6/1
  Demux/7 -> NOT7/1
  Demux/8 -> NOT8/1
  Demux1/1 -> NOT1/2
  Demux1/2 -> NOT2/2
  Demux1/3 -> NOT3/2
  Demux1/4 -> NOT4/2
  Demux1/5 -> NOT5/2
  Demux1/6 -> NOT6/2
  Demux1/7 -> NOT7/2
  Demux1/8 -> NOT8/2
  In1/1 -> Demux2/1, Demux/1
  In2/1 -> Demux1/1, Demux3/1
  NOT1/1 -> NOT9/1
  NOT2/1 -> NOT9/2
  NOT3/1 -> NOT9/3
  NOT4/1 -> NOT9/4
  NOT5/1 -> NOT9/5
  NOT6/1 -> NOT9/6
  NOT7/1 -> NOT9/7
  NOT8/1 -> NOT9/8
  NOT9/1 -> Logical Operator25/2, Out2/1
  Logical Operator14/1 -> Logical Operator16/3
  Logical Operator7/1 -> Logical Operator8/1
  Logical Operator13/1 -> Logical Operator15/1, Logical Operator6/3
  Demux3/1 -> Logical Operator9/1
  Demux2/2 -> Logical Operator8/2
  Logical Operator15/1 -> Logical Operator16/1
  Demux2/3 -> Logical Operator13/2
  Logical Operator10/1 -> Logical Operator8/3
  Logical Operator6/1 -> Logical Operator25/1, Out1/1
  Demux2/1 -> Logical Operator5/1
  Demux2/4 -> Logical Operator16/2
  Logical Operator11/1 -> Logical Operator13/3
  Logical Operator16/1 -> Logical Operator24/1, Logical Operator6/4
  Logical Operator9/1 -> Logical Operator5/2
  Demux3/2 -> Logical Operator10/1
  Logical Operator12/1 -> Logical Operator13/1
  Demux3/3 -> Logical Operator11/1
  Demux3/4 -> Logical Operator14/1
  Logical Operator5/1 -> Logical Operator7/1, Logical Operator6/1
  Logical Operator8/1 -> Logical Operator12/1, Logical Operator6/2
  Demux2/5 -> Logical Operator20/1
  Demux3/5 -> Logical Operator23/1
  Logical Operator17/1 -> Logical Operator19/3
  Logical Operator19/1 -> Logical Operator6/8
  Logical Operator1/1 -> Logical Operator22/3
  Logical Operator2/1 -> Logical Operator4/3
  Demux3/8 -> Logical Operator17/1
  Demux3/7 -> Logical Operator2/1
  Demux2/7 -> Logical Operator4/2
  Logical Operator3/1 -> Logical Operator4/1
  Logical Operator21/1 -> Logical Operator22/1
  Logical Operator22/1 -> Logical Operator6/6, Logical Operator3/1
  Demux2/8 -> Logical Operator19/2
  Logical Operator18/1 -> Logical Operator19/1
  Logical Operator20/1 -> Logical Operator6/5, Logical Operator21/1
  Demux3/6 -> Logical Operator1/1
  Logical Operator4/1 -> Logical Operator6/7, Logical Operator18/1
  Demux2/6 -> Logical Operator22/2
  Logical Operator24/1 -> Logical Operator20/2
  Logical Operator23/1 -> Logical Operator20/3
  Logical Operator25/1 -> Out3/1

== system bit32alu/Subsystem2/Comparartor/Comparator3 ==
  In1 : Inport
  In2 : Inport  Port=2
  Demux{,1..3} (4 alike) : Demux  Outputs=8
  Logical Operator{1..3,7,9..12,14..15,17..18,21,23..24} (15 alike) : Logic  Operator=NOT  Inputs=3  AllPortsSameDT=off  OutDataTypeStr=boolean
  Logical Operator{4,8,13,16,19..20,22} (7 alike) : Logic  Inputs=3  AllPortsSameDT=off  OutDataTypeStr=boolean
  Logical Operator25 : Logic  Operator=NOR  AllPortsSameDT=off  OutDataTypeStr=boolean
  Logical Operator5 : Logic  AllPortsSameDT=off  OutDataTypeStr=boolean
  Logical Operator6 : Logic  Operator=OR  Inputs=8  AllPortsSameDT=off  OutDataTypeStr=boolean
  NOT{1..8} (8 alike) : Logic  Operator=NXOR  AllPortsSameDT=off  OutDataTypeStr=boolean
  NOT9 : Logic  Inputs=8  AllPortsSameDT=off  OutDataTypeStr=boolean
  Out1 : Outport
  Out2 : Outport  Port=2
  Out3 : Outport  Port=3
  wires:
  Demux/1 -> NOT1/1
  Demux/2 -> NOT2/1
  Demux/3 -> NOT3/1
  Demux/4 -> NOT4/1
  Demux/5 -> NOT5/1
  Demux/6 -> NOT6/1
  Demux/7 -> NOT7/1
  Demux/8 -> NOT8/1
  Demux1/1 -> NOT1/2
  Demux1/2 -> NOT2/2
  Demux1/3 -> NOT3/2
  Demux1/4 -> NOT4/2
  Demux1/5 -> NOT5/2
  Demux1/6 -> NOT6/2
  Demux1/7 -> NOT7/2
  Demux1/8 -> NOT8/2
  In1/1 -> Demux2/1, Demux/1
  In2/1 -> Demux1/1, Demux3/1
  NOT1/1 -> NOT9/1
  NOT2/1 -> NOT9/2
  NOT3/1 -> NOT9/3
  NOT4/1 -> NOT9/4
  NOT5/1 -> NOT9/5
  NOT6/1 -> NOT9/6
  NOT7/1 -> NOT9/7
  NOT8/1 -> NOT9/8
  NOT9/1 -> Logical Operator25/2, Out2/1
  Logical Operator14/1 -> Logical Operator16/3
  Logical Operator7/1 -> Logical Operator8/1
  Logical Operator13/1 -> Logical Operator15/1, Logical Operator6/3
  Demux3/1 -> Logical Operator9/1
  Demux2/2 -> Logical Operator8/2
  Logical Operator15/1 -> Logical Operator16/1
  Demux2/3 -> Logical Operator13/2
  Logical Operator10/1 -> Logical Operator8/3
  Logical Operator6/1 -> Logical Operator25/1, Out1/1
  Demux2/1 -> Logical Operator5/1
  Demux2/4 -> Logical Operator16/2
  Logical Operator11/1 -> Logical Operator13/3
  Logical Operator16/1 -> Logical Operator24/1, Logical Operator6/4
  Logical Operator9/1 -> Logical Operator5/2
  Demux3/2 -> Logical Operator10/1
  Logical Operator12/1 -> Logical Operator13/1
  Demux3/3 -> Logical Operator11/1
  Demux3/4 -> Logical Operator14/1
  Logical Operator5/1 -> Logical Operator7/1, Logical Operator6/1
  Logical Operator8/1 -> Logical Operator12/1, Logical Operator6/2
  Demux2/5 -> Logical Operator20/1
  Demux3/5 -> Logical Operator23/1
  Logical Operator17/1 -> Logical Operator19/3
  Logical Operator19/1 -> Logical Operator6/8
  Logical Operator1/1 -> Logical Operator22/3
  Logical Operator2/1 -> Logical Operator4/3
  Demux3/8 -> Logical Operator17/1
  Demux3/7 -> Logical Operator2/1
  Demux2/7 -> Logical Operator4/2
  Logical Operator3/1 -> Logical Operator4/1
  Logical Operator21/1 -> Logical Operator22/1
  Logical Operator22/1 -> Logical Operator6/6, Logical Operator3/1
  Demux2/8 -> Logical Operator19/2
  Logical Operator18/1 -> Logical Operator19/1
  Logical Operator20/1 -> Logical Operator6/5, Logical Operator21/1
  Demux3/6 -> Logical Operator1/1
  Logical Operator4/1 -> Logical Operator6/7, Logical Operator18/1
  Demux2/6 -> Logical Operator22/2
  Logical Operator24/1 -> Logical Operator20/2
  Logical Operator23/1 -> Logical Operator20/3
  Logical Operator25/1 -> Out3/1

== system bit32alu/Subsystem2/Decrementer/Subtractor1 ==
  In1 : Inport
  In2 : Inport  Port=2
  Logical Operator2 : Logic  Operator=NOT  AllPortsSameDT=off  OutDataTypeStr=boolean
  Subtractor : Subsystem
  Zeros1 : Constant
  Out1 : Outport
  Out2 : Outport  Port=2
  wires:
  In2/1 -> Logical Operator2/1
  Subtractor/1(Out1) -> Out1/1
  In1/1 -> Subtractor/1(In1)
  Subtractor/2(Out2) -> Out2/1
  Logical Operator2/1 -> Subtractor/3(In3)
  Zeros1/1 -> Subtractor/2(In2)

== system bit32alu/Subsystem2/Incrementer/Incrementer ==
  In1 : Inport
  In2 : Inport  Port=2
  Subsystem : Subsystem
  Zeros1 : Constant  Value=0
  Out1 : Outport
  Out2 : Outport  Port=2
  wires:
  Subsystem/2(Out2) -> Out2/1
  In2/1 -> Subsystem/3(In3)
  Zeros1/1 -> Subsystem/2(In2)
  In1/1 -> Subsystem/1(In1)
  Subsystem/1(Out1) -> Out1/1

== system bit32alu/Subsystem2/Multiplier/Subsystem ==
  In1 : Inport
  In2 : Inport  Port=2
  In3 : Inport  Port=3
  Demux : Demux  Outputs=2
  Demux1 : Demux  Outputs=2
  Mux : Mux  Inputs=2
  Subsystem1 : Subsystem
  Subsystem2 : Subsystem
  Out1 : Outport
  Out2 : Outport  Port=2
  wires:
  Mux/1 -> Out2/1
  In3/1 -> Demux1/1
  Subsystem2/2(Out2) -> Mux/2
  In1/1 -> Demux/1
  Subsystem2/1(Out1) -> Subsystem1/2(In2)
  Subsystem1/2(Out2) -> Mux/1
  Demux1/2 -> Subsystem2/3(In3)
  In2/1 -> Subsystem2/2(In2)
  Demux/2 -> Subsystem2/1(In1)
  Subsystem1/1(Out1) -> Out1/1
  Demux1/1 -> Subsystem1/3(In3)
  Demux/1 -> Subsystem1/1(In1)

== system bit32alu/Subsystem2/Multiplier/Subsystem1 ==
  In1 : Inport
  In2 : Inport  Port=2
  Constant17 : Constant  Value=0
  Demux : Demux  Outputs=16
  Demux1 : Demux  Outputs=16
  Display1 : Display
  Logical Operator : Logic  Operator=XOR  AllPortsSameDT=off  OutDataTypeStr=boolean
  Logical Operator1 : Logic  AllPortsSameDT=off  OutDataTypeStr=boolean
  Mux : Mux  Inputs=16
  Mux1 : Mux  Inputs=16
  Subsystem : Subsystem
  Subsystem1 : Subsystem
  Subsystem2 : Subsystem
  Subsystem3 : Subsystem
  Subsystem4 : Subsystem
  Subsystem5 : Subsystem
  Subsystem6 : Subsystem
  Out1 : Outport
  Out2 : Outport  Port=2
  wires:
  Subsystem3/11(Out11) -> Subsystem/27(In27)
  Subsystem5/16(Out16) -> Mux1/7
  Subsystem/16(Out16) -> Subsystem5/15(In23)
  Subsystem5/7(Out7) -> Subsystem6/30(In30)
  Subsystem2/14(Out14) -> Subsystem/14(In22)
  Subsystem4/9(Out9) -> Mux1/9
  Subsystem5/11(Out11) -> Mux1/2
  Subsystem2/15(Out15) -> Subsystem/15(In23)
  Subsystem3/16(Out16) -> Subsystem/32(In32)
  Subsystem3/6(Out6) -> Subsystem/22(In14)
  Subsystem6/10(Out10) -> Mux/9
  Subsystem5/2(Out2) -> Subsystem6/25(In25)
  Subsystem4/7(Out7) -> Subsystem5/31(In31)
  Subsystem2/11(Out11) -> Subsystem/11(In19)
  Subsystem3/9(Out9) -> Subsystem/25(In25)
  Subsystem1/2(Out2) -> Subsystem6/2(In2)
  Subsystem1/3(Out3) -> Subsystem6/3(In3)
  Subsystem/17(Out17) -> Subsystem5/16(In24)
  Subsystem/4(Out4) -> Subsystem5/3(In3)
  Subsystem3/8(Out8) -> Subsystem/24(In16)
  Subsystem/11(Out11) -> Subsystem5/10(In18)
  Logical Operator1/1 -> Subsystem6/23(In15)
  Subsystem3/2(Out2) -> Subsystem/18(In10)
  Subsystem1/13(Out13) -> Subsystem6/13(14)
  Subsystem4/4(Out4) -> Subsystem5/28(In28)
  Subsystem5/17(Out17) -> Mux1/8
  Subsystem5/5(Out5) -> Subsystem6/28(In28)
  Subsystem1/8(Out8) -> Subsystem6/8(In8)
  Subsystem2/3(Out3) -> Subsystem/3(In3)
  Subsystem5/6(Out6) -> Subsystem6/29(In29)
  Subsystem/2(Out2) -> Subsystem5/1(In1)
  Subsystem4/1(Out1) -> Subsystem5/25(In25)
  Subsystem1/7(Out7) -> Subsystem6/7(In7)
  Subsystem5/9(Out9) -> Subsystem6/32(In32)
  Subsystem6/8(Out8) -> Mux/7
  Subsystem1/5(Out5) -> Subsystem6/5(In5)
  Subsystem6/11(Out11) -> Mux/10
  Subsystem1/6(Out6) -> Subsystem6/6(In6)
  Subsystem/7(Out7) -> Subsystem5/6(In6)
  Subsystem2/16(Out16) -> Subsystem/16(In24)
  Demux/7 -> Subsystem2/7(In7), Subsystem1/7(In7)
  Demux1/14 -> Subsystem4/14(In14), Subsystem2/14(In14)
  Demux/16 -> Subsystem4/8(In8), Subsystem3/8(In8)
  Subsystem2/1(Out1) -> Subsystem/1(In1)
  Subsystem5/15(Out15) -> Mux1/6
  Subsystem4/16(Out16) -> Mux1/16
  Subsystem3/4(Out4) -> Subsystem/20(In12)
  Subsystem/1(Out1) -> Logical Operator1/2, Logical Operator/2
  Subsystem1/4(Out4) -> Subsystem6/4(In4)
  Subsystem4/11(Out11) -> Mux1/11
  Demux/1 -> Subsystem1/1(In1), Subsystem2/1(In1)
  Subsystem3/10(Out10) -> Subsystem/26(In26)
  Subsystem6/2(Out2) -> Mux/1
  Subsystem/9(Out9) -> Subsystem5/8(In8)
  Demux1/3 -> Subsystem3/11(In11), Subsystem1/11(In11)
  Demux1/7 -> Subsystem3/15(In15), Subsystem1/15(In15)
  Subsystem/5(Out5) -> Subsystem5/4(In4)
  Mux/1 -> Out1/1
  Subsystem5/10(Out10) -> Mux1/1
  Subsystem1/12(Out12) -> Subsystem6/12(In20)
  Subsystem2/6(Out6) -> Subsystem/6(In6)
  Demux/13 -> Subsystem4/5(In5), Subsystem3/5(In5)
  Demux/10 -> Subsystem4/2(In2), Subsystem3/2(In2)
  Demux/11 -> Subsystem4/3(In3), Subsystem3/3(In3)
  Subsystem1/11(Out11) -> Subsystem6/11(In19)
  Subsystem6/17(Out17) -> Mux/16
  Demux/9 -> Subsystem4/1(In1), Subsystem3/1(In1)
  Subsystem4/15(Out15) -> Mux1/15
  Subsystem5/8(Out8) -> Subsystem6/31(In31)
  Demux1/1 -> Subsystem1/9(In9), Subsystem3/9(In9)
  Demux1/2 -> Subsystem3/10(In10), Subsystem1/10(In10)
  Demux/8 -> Subsystem2/8(In8), Subsystem1/8(In8)
  Demux/14 -> Subsystem4/6(In6), Subsystem3/6(In6)
  Subsystem1/15(Out15) -> Subsystem6/15(In23)
  Demux1/9 -> Subsystem2/9(In9), Subsystem4/9(In9)
  Subsystem5/14(Out14) -> Mux1/5
  Demux/6 -> Subsystem1/6(In6), Subsystem2/6(In6)
  Subsystem2/7(Out7) -> Subsystem/7(In7)
  Subsystem2/4(Out4) -> Subsystem/4(In4)
  Demux1/5 -> Subsystem3/13(In13), Subsystem1/13(In13)
  Subsystem/8(Out8) -> Subsystem5/7(In7)
  Logical Operator/1 -> Subsystem6/24(In16)
  Demux1/12 -> Subsystem2/12(In12), Subsystem4/12(In12)
  Subsystem2/9(Out9) -> Subsystem/9(In17)
  Subsystem5/13(Out13) -> Mux1/4
  Subsystem5/3(Out3) -> Subsystem6/26(In26)
  Demux1/8 -> Subsystem1/16(In16), Subsystem3/16(In16)
  Subsystem4/14(Out14) -> Mux1/14
  Constant17/1 -> Subsystem5/24(In16), Subsystem5/23(In15), Subsystem5/22(In14), Subsystem5/21(In13), Subsystem5/20(In12), Subsystem5/19(In11), Subsystem5/18(In10), Subsystem5/17(In9), Subsystem6/17(In9), Subsystem6/18(In10), Subsystem6/20(In12), Subsystem6/21(In13), Subsystem6/22(In14), Subsystem6/19(In11)
  Subsystem3/13(Out13) -> Subsystem/29(In29)
  Subsystem1/16(Out16) -> Subsystem6/16(In24)
  Subsystem/15(Out15) -> Subsystem5/14(In22)
  Demux1/13 -> Subsystem2/13(In13), Subsystem4/13(In13)
  Subsystem/12(Out12) -> Subsystem5/11(In19)
  Demux1/16 -> Subsystem2/16(In16), Subsystem4/16(In16)
  Subsystem5/12(Out12) -> Mux1/3
  Subsystem3/15(Out15) -> Subsystem/31(In31)
  Subsystem6/9(Out9) -> Mux/8
  Demux/5 -> Subsystem1/5(In5), Subsystem2/5(In5)
  Subsystem6/4(Out4) -> Mux/3
  Subsystem6/3(Out3) -> Mux/2
  Subsystem4/13(Out13) -> Mux1/13
  Demux1/6 -> Subsystem3/14(In14), Subsystem1/14(In14)
  Subsystem/6(Out6) -> Subsystem5/5(In5)
  Subsystem/13(Out13) -> Subsystem5/12(In20)
  Subsystem6/13(Out13) -> Mux/12
  Subsystem6/12(Out12) -> Mux/11
  Subsystem4/10(Out10) -> Mux1/10
  Subsystem3/5(Out5) -> Subsystem/21(In13)
  Subsystem/10(Out10) -> Subsystem5/9(In17)
  Subsystem2/12(Out12) -> Subsystem/12(In20)
  Subsystem5/1(Out1) -> Logical Operator/1, Logical Operator1/1
  Subsystem6/5(Out5) -> Mux/4
  Subsystem3/1(Out1) -> Subsystem/17(In9)
  Subsystem4/8(Out8) -> Subsystem5/32(In32)
  Subsystem3/12(Out12) -> Subsystem/28(In28)
  Subsystem6/1(Out1) -> Display1/1
  Subsystem4/6(Out6) -> Subsystem5/30(In30)
  Subsystem2/2(Out2) -> Subsystem/2(In2)
  Subsystem2/10(Out10) -> Subsystem/10(In18)
  Subsystem4/5(Out5) -> Subsystem5/29(In29)
  Subsystem2/13(Out13) -> Subsystem/13(14)
  Subsystem1/1(Out1) -> Subsystem6/1(In1)
  Subsystem6/7(Out7) -> Mux/6
  Subsystem6/14(Out14) -> Mux/13
  Subsystem5/4(Out4) -> Subsystem6/27(In27)
  Subsystem2/8(Out8) -> Subsystem/8(In8)
  Subsystem/14(Out14) -> Subsystem5/13(14)
  Subsystem6/16(Out16) -> Mux/15
  Demux/4 -> Subsystem2/4(In4), Subsystem1/4(In4)
  Subsystem1/10(Out10) -> Subsystem6/10(In18)
  Demux/12 -> Subsystem4/4(In4), Subsystem3/4(In4)
  Subsystem3/14(Out14) -> Subsystem/30(In30)
  Subsystem2/5(Out5) -> Subsystem/5(In5)
  Demux1/10 -> Subsystem2/10(In10), Subsystem4/10(In10)
  Demux/2 -> Subsystem1/2(In2), Subsystem2/2(In2)
  Subsystem6/6(Out6) -> Mux/5
  Subsystem/3(Out3) -> Subsystem5/2(In2)
  Subsystem4/12(Out12) -> Mux1/12
  Demux1/4 -> Subsystem1/12(In12), Subsystem3/12(In12)
  Demux/15 -> Subsystem4/7(In7), Subsystem3/7(In7)
  Subsystem1/14(Out14) -> Subsystem6/14(In22)
  Subsystem3/3(Out3) -> Subsystem/19(In11)
  Subsystem6/15(Out15) -> Mux/14
  Subsystem1/9(Out9) -> Subsystem6/9(In17)
  Demux1/11 -> Subsystem2/11(In11), Subsystem4/11(In11)
  Subsystem4/2(Out2) -> Subsystem5/26(In26)
  Demux/3 -> Subsystem1/3(In3), Subsystem2/3(In3)
  Subsystem4/3(Out3) -> Subsystem5/27(In27)
  Subsystem3/7(Out7) -> Subsystem/23(In15)
  Demux1/15 -> Subsystem2/15(In15), Subsystem4/15(In15)
  In1/1 -> Demux/1
  In2/1 -> Demux1/1
  Mux1/1 -> Out2/1
